simulink model "mpc_control_variable_kalman_observer"  (R2020b)
settings: Solver=VariableStepAuto  StartTime=0.0  StopTime=50  RelTol=1e-3
undefined symbols (not defined in the file): A, B, C, C_discrete, D, D_discrete, DiscIntNeverNeededParam, G, Gamma, h, h_plant, N, n, Phi, Q, Q0, Q1, Q2, R, reference, sat_max, sat_min, wind_final_value, wind_initial_value, wind_steptime, x0
settings Model: Creator=lucas  LastModifiedBy=lucas

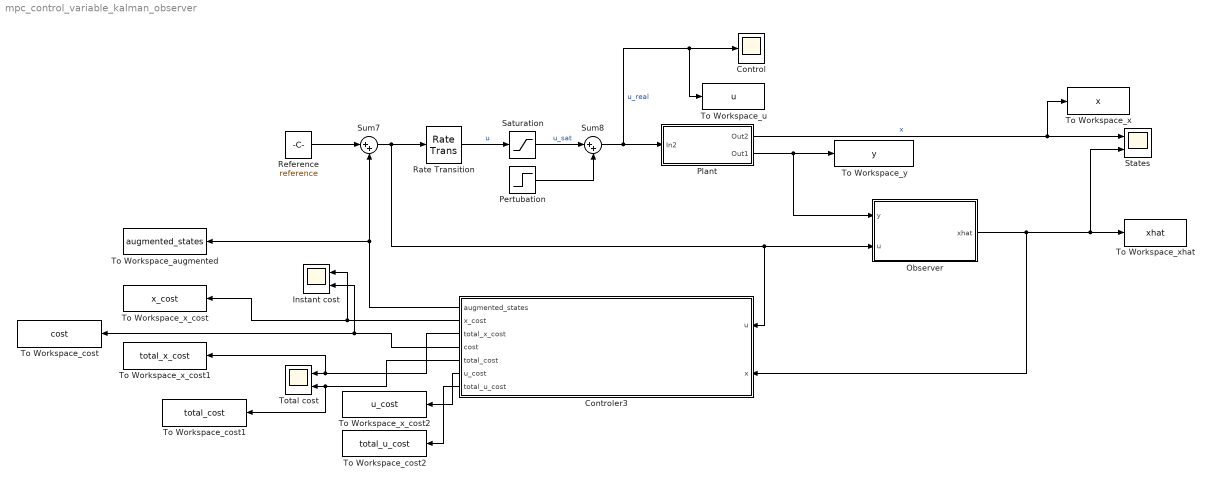
== system mpc_control_variable_kalman_observer ==
  Control : Scope
  Controler3 : Subsystem
  Instant cost : Scope  NumInputPorts=2
  Observer : Subsystem
  Pertubation : Step  Time=wind_steptime  Before=wind_initial_value  After=wind_final_value  SampleTime=h_plant
  Plant : Subsystem
  Rate Transition : RateTransition  Integrity=off  OutPortSampleTimeMultiple=0.01  OutPortSampleTime=h_plant
  Reference : Constant  Value=reference  SampleTime=h
  Saturation : Saturate  UpperLimit=sat_max  LowerLimit=sat_min
  States : Scope  NumInputPorts=2
  Sum7 : Sum  Inputs=|++
  Sum8 : Sum  Inputs=|++
  To Workspace_augmented : ToWorkspace  VariableName=augmented_states  SaveFormat=Timeseries  SampleTime=-1
  To Workspace_cost : ToWorkspace  VariableName=cost  SaveFormat=Timeseries  SampleTime=-1
  To Workspace_cost1 : ToWorkspace  VariableName=total_cost  SaveFormat=Timeseries  SampleTime=-1
  To Workspace_cost2 : ToWorkspace  VariableName=total_u_cost  SaveFormat=Timeseries  SampleTime=-1
  To Workspace_u : ToWorkspace  VariableName=u  SaveFormat=Timeseries  SampleTime=-1
  To Workspace_x : ToWorkspace  VariableName=x  SaveFormat=Timeseries  SampleTime=-1
  To Workspace_x_cost : ToWorkspace  VariableName=x_cost  SaveFormat=Timeseries  SampleTime=-1
  To Workspace_x_cost1 : ToWorkspace  VariableName=total_x_cost  SaveFormat=Timeseries  SampleTime=-1
  To Workspace_x_cost2 : ToWorkspace  VariableName=u_cost  SaveFormat=Timeseries  SampleTime=-1
  To Workspace_xhat : ToWorkspace  VariableName=xhat  SaveFormat=Timeseries  SampleTime=-1
  To Workspace_y : ToWorkspace  VariableName=y  SaveFormat=Timeseries  SampleTime=-1
  Total cost : Scope  NumInputPorts=2
  wires:
  Sum8/1 -> Plant/1(In2), To Workspace_u/1, Control/1  "u_real"
  Plant/1(Out2) -> To Workspace_x/1, States/1  "x"
  Controler3/1(augmented_states) -> To Workspace_augmented/1, Sum7/2
  Reference/1 -> Sum7/1
  Pertubation/1 -> Sum8/2
  Saturation/1 -> Sum8/1  "u_sat"
  Observer/1(xhat) -> Controler3/2(x), To Workspace_xhat/1, States/2
  Sum7/1 -> Controler3/1(u), Observer/2(u), Rate Transition/1
  Plant/2(Out1) -> Observer/1(y), To Workspace_y/1
  Rate Transition/1 -> Saturation/1  "u"
  Controler3/2(x_cost) -> To Workspace_x_cost/1, Instant cost/1
  Controler3/4(cost) -> To Workspace_cost/1, Instant cost/2
  Controler3/5(total_cost) -> To Workspace_cost1/1, Total cost/2
  Controler3/3(total_x_cost) -> To Workspace_x_cost1/1, Total cost/1
  Controler3/7(total_u_cost) -> To Workspace_cost2/1
  Controler3/6(u_cost) -> To Workspace_x_cost2/1

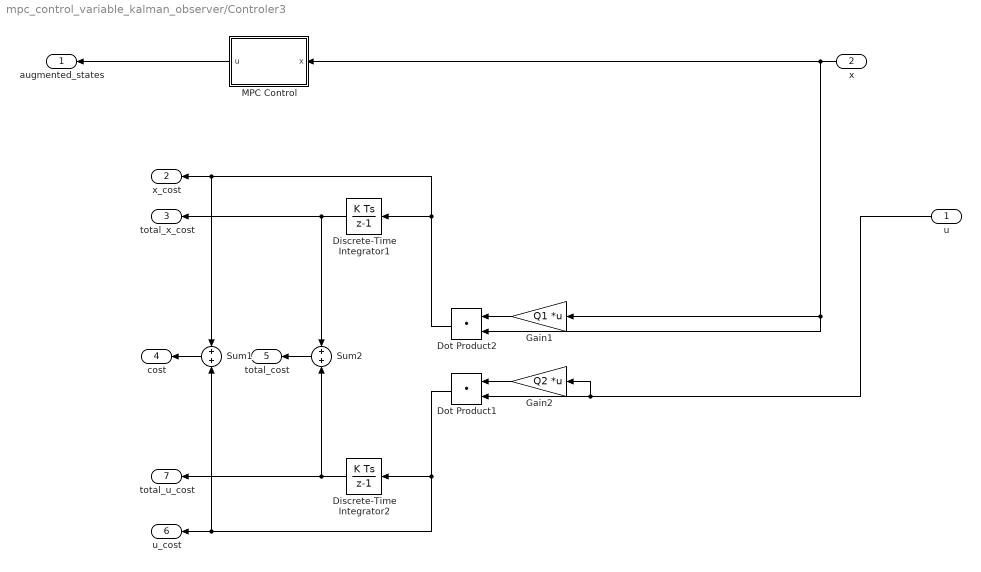
== system mpc_control_variable_kalman_observer/Controler3 ==
  u : Inport
  x : Inport  Port=2
  Discrete-Time Integrator1 : DiscreteIntegrator  SampleTime=-1  ICPrevOutput=DiscIntNeverNeededParam  ICPrevScaledInput=DiscIntNeverNeededParam
  Discrete-Time Integrator2 : DiscreteIntegrator  SampleTime=-1  ICPrevOutput=DiscIntNeverNeededParam  ICPrevScaledInput=DiscIntNeverNeededParam
  Dot Product1 : DotProduct  InputSameDT=on  OutDataTypeStr=Inherit: Inherit via internal rule
  Dot Product2 : DotProduct  InputSameDT=on  OutDataTypeStr=Inherit: Inherit via internal rule
  Gain1 : Gain  Gain=Q1  Multiplication=Matrix(K*u)
  Gain2 : Gain  Gain=Q2  Multiplication=Matrix(K*u)
  MPC Control : MATLAB Function  TreatAsAtomicUnit=on
  Sum1 : Sum  Inputs=+|+
  Sum2 : Sum  Inputs=+|+
  augmented_states : Outport
  x_cost : Outport  Port=2
  total_x_cost : Outport  Port=3
  cost : Outport  Port=4
  total_cost : Outport  Port=5
  u_cost : Outport  Port=6
  total_u_cost : Outport  Port=7
  wires:
  Gain1/1 -> Dot Product2/1
  u/1 -> Dot Product1/2, Gain2/1
  Dot Product2/1 -> Sum1/1, x_cost/1, Discrete-Time Integrator1/1
  MPC Control/1(u) -> augmented_states/1
  Gain2/1 -> Dot Product1/1
  x/1 -> MPC Control/1(x), Dot Product2/2, Gain1/1
  Dot Product1/1 -> Discrete-Time Integrator2/1, Sum1/2, u_cost/1
  Discrete-Time Integrator1/1 -> total_x_cost/1, Sum2/1
  Discrete-Time Integrator2/1 -> Sum2/2, total_u_cost/1
  Sum1/1 -> cost/1
  Sum2/1 -> total_cost/1

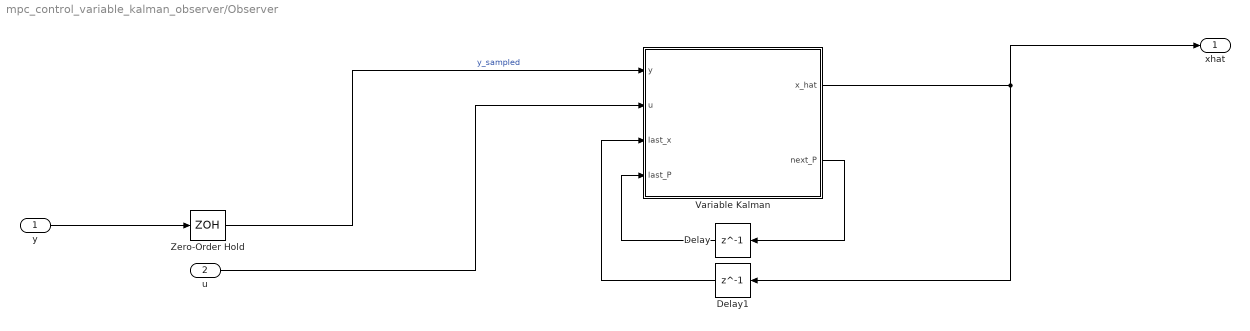
== system mpc_control_variable_kalman_observer/Observer ==
  y : Inport
  u : Inport  Port=2
  Delay : Delay  DelayLength=1  InitialCondition=eye(n)  SampleTime=h
  Delay1 : Delay  DelayLength=1  InitialCondition=zeros(n,1)  SampleTime=h
  Variable Kalman : MATLAB Function  TreatAsAtomicUnit=on
  Zero-Order Hold : ZeroOrderHold  SampleTime=h
  xhat : Outport
  wires:
  Zero-Order Hold/1 -> Variable Kalman/1(y)  "y_sampled"
  y/1 -> Zero-Order Hold/1
  u/1 -> Variable Kalman/2(u)
  Variable Kalman/1(x_hat) -> Delay1/1, xhat/1
  Variable Kalman/2(next_P) -> Delay/1
  Delay/1 -> Variable Kalman/4(last_P)
  Delay1/1 -> Variable Kalman/3(last_x)

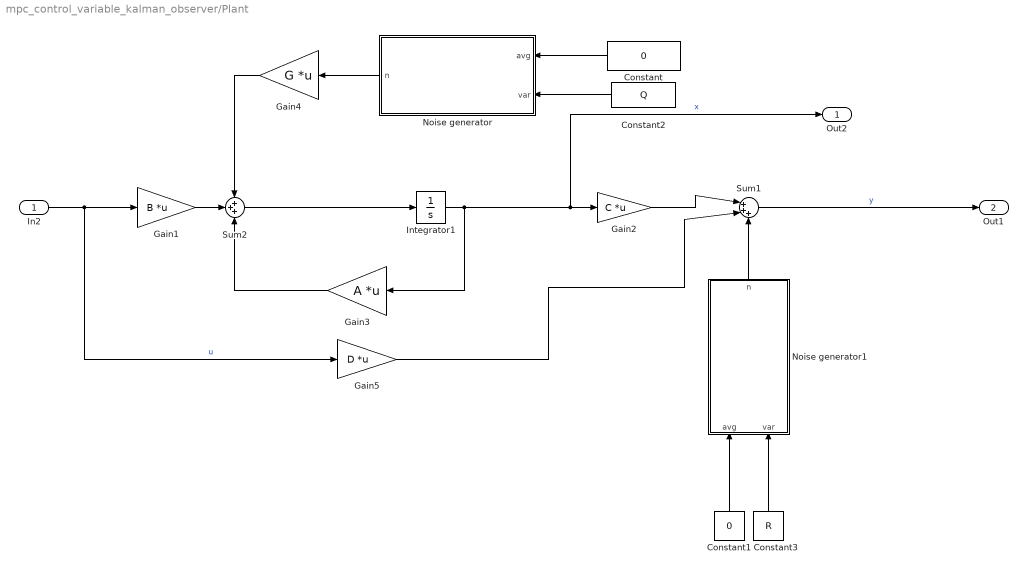
== system mpc_control_variable_kalman_observer/Plant ==
  In2 : Inport
  Constant : Constant  Value=0  VectorParams1D=off
  Constant1 : Constant  Value=0
  Constant2 : Constant  Value=Q
  Constant3 : Constant  Value=R
  Gain1 : Gain  Gain=B  Multiplication=Matrix(K*u) (u vector)
  Gain2 : Gain  Gain=C  Multiplication=Matrix(K*u) (u vector)
  Gain3 : Gain  Gain=A  Multiplication=Matrix(K*u) (u vector)
  Gain4 : Gain  Gain=G  Multiplication=Matrix(K*u) (u vector)
  Gain5 : Gain  Gain=D  Multiplication=Matrix(K*u) (u vector)
  Integrator1 : Integrator  InitialCondition=x0
  Noise generator : MATLAB Function  TreatAsAtomicUnit=on
  Noise generator1 : MATLAB Function  TreatAsAtomicUnit=on
  Sum1 : Sum  Inputs=|+++
  Sum2 : Sum  Inputs=+++
  Out2 : Outport
  Out1 : Outport  Port=2
  wires:
  Sum2/1 -> Integrator1/1
  Gain2/1 -> Sum1/1
  Sum1/1 -> Out1/1  "y"
  In2/1 -> Gain5/1, Gain1/1  "u"
  Integrator1/1 -> Gain3/1, Out2/1, Gain2/1  "x"
  Gain1/1 -> Sum2/2
  Gain3/1 -> Sum2/3
  Noise generator/1(n) -> Gain4/1
  Gain4/1 -> Sum2/1
  Constant/1 -> Noise generator/1(avg)
  Constant1/1 -> Noise generator1/1(avg)
  Constant3/1 -> Noise generator1/2(var)
  Constant2/1 -> Noise generator/2(var)
  Noise generator1/1(n) -> Sum1/3
  Gain5/1 -> Sum1/2

== matlab function mpc_control_variable_kalman_observer/Plant/Noise generator1 ==
  data: avg input; n output; var input
function n = generate_gaussian_noise(avg, var)
n = avg + var*randn(length(var), 1);

== matlab function mpc_control_variable_kalman_observer/Controler3/MPC Control ==
  settings: updateMethod=DISCRETE  sampleTime=h
  data: Q1 parameter; Q2 parameter; Q0 parameter; n parameter; Phi parameter; Gamma parameter; x input; N parameter; u output
function u  = mpc(Q1,Q2,Q0,n,Phi,Gamma,x,N)
%#codegen

tStart = tic;

coder.extrinsic('quadprog');

U = zeros(N,1);
Gain = zeros(2,1);
fval = 0;
z = zeros(N,1);

M0 = [Phi];
coder.varsize("Mu");
Mu = [Gamma, zeros(size(Gamma,1), N-1)];
Mu_aux = Mu;
Qtil =  kron(eye((N-1)*(n-1)), Q1);
Rbar = kron(eye(N*size(Gamma,2)), Q2);
Qbar = blkdiag(Qtil, Q0);
for i = 1:N-1
    M0 = [M0; Phi^(i+1)];
end
for i = 1:N-1
    Mu_aux = [Mu_aux(1)*Gamma, Mu_aux(:,1:length(Mu_aux)-1)];
    Mu = [Mu; Mu_aux];
end
Qxo = Q1 + M0'*Qbar*M0;
Qu = 2*Mu'*Qbar*Mu + Rbar;
Qxu = 2*M0'*Qbar*Mu;


[U , fval] = quadprog(2*Qu, 2*Qxu'*x);%, G_teste, W_teste + S_teste*x);
u = U(1,:);

tEnd = toc(tStart);

== matlab function mpc_control_variable_kalman_observer/Observer/Variable Kalman ==
  data: y input; u input; last_x input; last_P input; x_hat output; next_P output; Gamma parameter; Phi parameter; C_discrete parameter; R parameter; G parameter; Q parameter; D_discrete parameter
function [x_hat, next_P] = fcn(y, u, last_x, last_P, Gamma, Phi, C_discrete, R, G, Q, D_discrete)

    P = inv(last_P) + C_discrete'*inv(R)*C_discrete;
    P = inv(P);
    next_P = Phi*P*Phi' + G*Q*G';
    L = P*C_discrete'*inv(R);
    x = last_x + L*(y - C_discrete*last_x - D_discrete*u);
    x_hat = Phi*x + Gamma*u;

== matlab function mpc_control_variable_kalman_observer/Plant/Noise generator ==
  data: avg input; n output; var input
function n = generate_gaussian_noise(avg, var)
n = avg + var*randn(length(var), 1);
